simulink model "segway"  (R2018b)
settings: Solver=FixedStepDiscrete  StartTime=0.0  StopTime=inf  FixedStep=0.02  RelTol=1e-3  EnableMultiTasking=on
libraries: simulink x1, arduinolib x1
settings Model: SimulationMode=external  ExtModeTrigDuration=2  Creator=root  LastModifiedBy=root
settings OptimizationCC: EnhancedBackFolding=on  PassReuseOutputArgsAs=Individual arguments  MaxStackSize=64  OptimizeBlockOrder=speed  DifferentSizesBufferReuse=on  OptimizationCustomize=off
settings DebuggingCC: ParameterTunabilityLossMsg=error
settings HardwareCC: ProdBitPerInt=16  ProdBitPerPointer=16  ProdBitPerSizeT=16  ProdBitPerPtrDiffT=16  ProdLargestAtomicFloat=None  ProdWordSize=8  ProdHWDeviceType=Atmel->AVR
settings SFSimCC: MATLABDynamicMemAlloc=off
settings RTWCC: SystemTargetFile=ert.tlc  HardwareBoard=Arduino Mega 2560  TemplateMakefile=ert_default_tmf  GenerateReport=on  Toolchain=Arduino AVR  BuildConfiguration=Faster Runs  IncludeHyperlinkInReport=on  LaunchReport=on  GenerateTraceInfo=on  GenerateTraceReport=on  GenerateTraceReportSl=on  GenerateTraceReportSf=on  GenerateTraceReportEml=on
settings CodeAppCC: ForceParamTrailComments=on  IgnoreCustomStorageClasses=off  OperatorAnnotations=on  SimulinkDataObjDesc=on  SFDataObjDesc=on  InsertBlockDesc=on
settings ERTTargetCC: SupportContinuousTime=on  SupportVariableSizeSignals=on

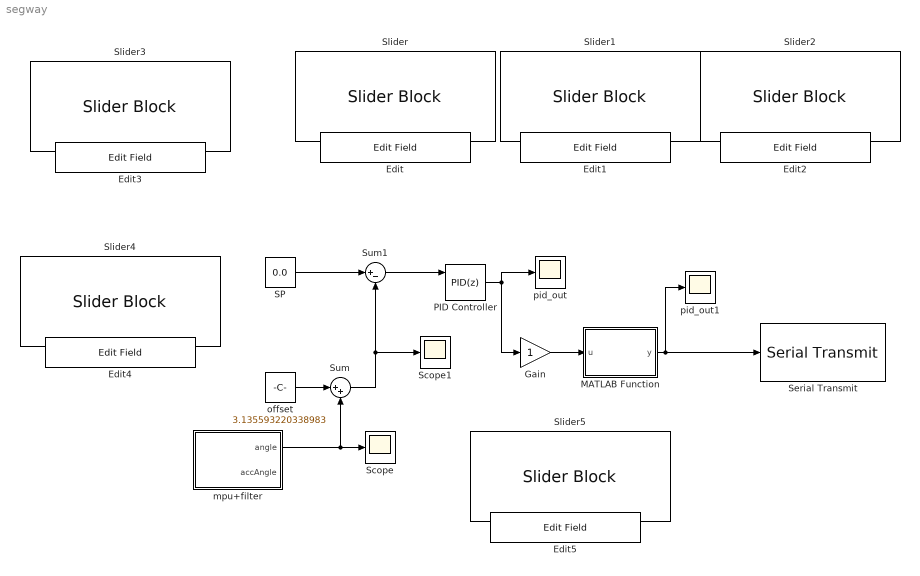
== system segway ==
  Edit : EditField  WebBlockId=59  LabelPosition=Hide  ShowInitialText=on  Alignment=Center
  Edit1 : EditField  WebBlockId=60  LabelPosition=Hide  ShowInitialText=on  Alignment=Center
  Edit2 : EditField  WebBlockId=61  LabelPosition=Hide  ShowInitialText=on  Alignment=Center
  Edit3 : EditField  WebBlockId=63  LabelPosition=Hide  ShowInitialText=on  Alignment=Center
  Edit4 : EditField  WebBlockId=65  LabelPosition=Hide  ShowInitialText=on  Alignment=Center
  Edit5 : EditField  WebBlockId=67  LabelPosition=Hide  ShowInitialText=on  Alignment=Center
  Gain : Gain
  MATLAB Function : MATLAB Function  TreatAsAtomicUnit=on
  PID Controller : simulink/Continuous/PID Controller  Controller=PID  Form=Parallel  TimeDomain=Discrete-time  SampleTime=-1  IntegratorMethod=Forward Euler  FilterMethod=Forward Euler  ControllerParametersSource=internal  P=13.30508474576271  I=1.864406779661017  D=2.415254237288135  UseFilter=on  N=10  TunerSelectOption=Transfer Function Based (PID Tuner App)  InitialConditionSource=internal  InitialConditionForIntegrator=0  InitialConditionForFilter=0  DifferentiatorICPrevScaledInput=0  ExternalReset=rising  IgnoreLimit=on  TrackingMode=off  Kt=1  LimitOutput=on  UpperSaturationLimit=127  LowerSaturationLimit=-127  LinearizeAsGain=on  AntiWindupMode=clamping  Kb=1  POutMin=[]  POutMax=[]  IOutMin=[]  IOutMax=[]  DOutMin=[]  DOutMax=[]  NOutMin=[]  NOutMax=[]  SumOutMin=[]  SumOutMax=[]  SaturationOutMin=[]  SaturationOutMax=[]  PParamMin=[]  PParamMax=[]  IParamMin=[]  IParamMax=[]  DParamMin=[]  DParamMax=[]  NParamMin=[]  NParamMax=[]  KbParamMin=[]  KbParamMax=[]  KtParamMin=[]  KtParamMax=[]  KbOutMin=[]  KbOutMax=[]  KtOutMin=[]  KtOutMax=[]  IntegratorOutMin=[]  IntegratorOutMax=[]  FilterOutMin=[]  FilterOutMax=[]  SumI1OutMin=[]  SumI1OutMax=[]  SumI2OutMin=[]  SumI2OutMax=[]  SumI3OutMin=[]  SumI3OutMax=[]  SumI4OutMin=[]  SumI4OutMax=[]  SumDOutMin=[]  SumDOutMax=[]  DifferentiatorOutMin=[]  DifferentiatorOutMax=[]  FilterDiffOutCoefMin=[]  FilterDiffOutCoefMax=[]  ReciprocalOutMin=[]  ReciprocalOutMax=[]  SumDenOutMin=[]  SumDenOutMax=[]  SumNumOutMin=[]  SumNumOutMax=[]  DivideOutMin=[]  DivideOutMax=[]  IntegratorContinuousStateAttributes=''  IntegratorStateMustResolveToSignalObject=off  IntegratorRTWStateStorageClass=Auto  FilterContinuousStateAttributes=''  FilterStateMustResolveToSignalObject=off  FilterRTWStateStorageClass=Auto  ParallelPVariant=InternalParameters  IdealPVariant=Disabled  IVariant=InternalParameters  DVariant=InternalParameters  IntegratorVariant=Discrete  SatVariant=Enabled  AWVariant=DiscClampingParallel  PCopyVariant=Disabled  TRVariant=Disabled  FdbkBlocksVariant=Forward  IdealPFdbkVariant=Disabled  SatFdbkVariant=Disabled  DerivativeFilterVariant=ForwardEulerFilter  NVariant=InternalParameters  NCopyVariant=Disabled  FilterICVariant=InternalICsFilter  IntegratorICVariant=InternalICs  ExternalResetVariant=ExternalReset  TRSumVariant=Passthrough  SumFdbkVariant=Disabled  SumVariant=Sum_PID
  SP : Constant  Value=0.0
  Scope : Scope
  Scope1 : Scope
  Serial Transmit : arduinolib/Serial Transmit  portNumber=2  sendmode=write  label=y  sendformat=Decimal  floatprecision=2  blockPlatform=arduino
      settings: SourceProductName=Simulink Support Package for Arduino Hardware
  Slider : SliderBlock  WebBlockId=52  ScaleMax=20
  Slider1 : SliderBlock  WebBlockId=53  ScaleMax=5
  Slider2 : SliderBlock  WebBlockId=54  ScaleMax=5
  Slider3 : SliderBlock  WebBlockId=64  ScaleMax=20
  Slider4 : SliderBlock  WebBlockId=66  ScaleMax=20
  Slider5 : SliderBlock  WebBlockId=68  ScaleMax=5
  Sum : Sum  Inputs=|++
  Sum1 : Sum  Inputs=|+-
  mpu+filter : Subsystem
  offset : Constant  Value=3.135593220338983
  pid_out : Scope
  pid_out1 : Scope
  wires:
  mpu+filter/1(angle) -> Sum/2, Scope/1
  offset/1 -> Sum/1
  SP/1 -> Sum1/1
  Sum1/1 -> PID Controller/1
  PID Controller/1 -> pid_out/1, Gain/1
  MATLAB Function/1(y) -> pid_out1/1, Serial Transmit/1
  Gain/1 -> MATLAB Function/1(u)
  Sum/1 -> Scope1/1, Sum1/2

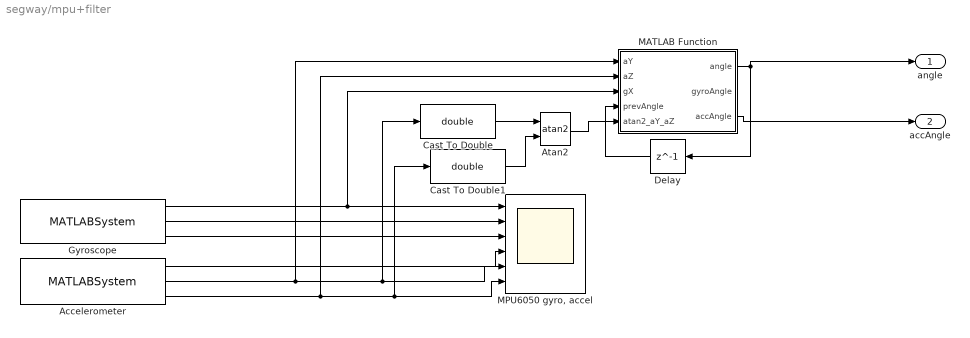
== system segway/mpu+filter ==
  Accelerometer : MATLABSystem  System=soMPU6050Accel  SimulateUsing=Code generation
      mask Type: soMPU6050Accel
      mask Display:
      | disp('soMPU6050Accel');
      | port_label('output',1,'xaccel');
      | port_label('output',2,'yaccel');
      | port_label('output',3,'zaccel');
  Atan2 : Trigonometry  Operator=atan2
  Cast To Double : DataTypeConversion  OutDataTypeStr=double
  Cast To Double1 : DataTypeConversion  OutDataTypeStr=double
  Delay : Delay  DelayLength=1  InitialCondition=0
  Gyroscope : MATLABSystem  System=soMPU6050Gyro  DLPFmode=0
      mask Type: soMPU6050Gyro
      mask Display:
      | disp('soMPU6050Gyro');
      | port_label('output',1,'xvel');
      | port_label('output',2,'yvel');
      | port_label('output',3,'zvel');
  MATLAB Function : MATLAB Function  TreatAsAtomicUnit=on
  "MPU6050 gyro, accel" : Scope  NumInputPorts=6
  angle : Outport
  accAngle : Outport  Port=2
  wires:
  Accelerometer/1 -> "MPU6050 gyro, accel"/4
  Gyroscope/3 -> "MPU6050 gyro, accel"/3
  Accelerometer/3 -> MATLAB Function/2(aZ), Cast To Double1/1, "MPU6050 gyro, accel"/6
  Accelerometer/2 -> MATLAB Function/1(aY), Cast To Double/1, "MPU6050 gyro, accel"/5
  Cast To Double/1 -> Atan2/1
  MATLAB Function/3(accAngle) -> accAngle/1
  Delay/1 -> MATLAB Function/4(prevAngle)
  Atan2/1 -> MATLAB Function/5(atan2_aY_aZ)
  MATLAB Function/1(angle) -> angle/1, Delay/1
  Gyroscope/1 -> MATLAB Function/3(gX), "MPU6050 gyro, accel"/1
  Gyroscope/2 -> "MPU6050 gyro, accel"/2
  Cast To Double1/1 -> Atan2/2

== matlab function segway/MATLAB Function ==
  data: u input; y output
function y = fcn(u)
if(u>0)
    u=u+5;
elseif(u<-5)
    u=u-5;
end

if(u>127)
    u=127;
elseif(u<-127)
    u=-127;
end

y = uint8(u + 127) ;

%y = [y 123]

== matlab function segway/mpu+filter/MATLAB Function ==
  data: aY input; angle output; aZ input; gX input; prevAngle input; atan2_aY_aZ input; gyroAngle output; accAngle output
function [angle , gyroAngle , accAngle]= fcn(aY , aZ , gX , prevAngle , atan2_aY_aZ )
  RAD_TO_DEG = 180.0/pi;
  sampleTime = 0.02;
  accAngle = atan2_aY_aZ*RAD_TO_DEG;
    
  % gyroRate = map(gX, -32768, 32767, -250, 250);
  gyroRate = double(gX)*(500) / (32767 + 32768);
  
  gyroAngle = double(gyroRate)*sampleTime;  
  %gyroAngle = double(gyroAngle )+ gyroRate*sampleTime/1000000.0;
  currentAngle = 0.9934*(prevAngle + gyroAngle) + 0.0066*(accAngle);
  angle = double(currentAngle);
